simulink model "TrayectoriaStateflow"  (R2023b)
settings: Solver=FixedStepDiscrete  StartTime=0.0  StopTime=inf  FixedStep=0.01  RelTol=1e-3  EnableMultiTasking=on
settings Model: ExtModeTrigDuration=2  Creator=Usuario_UMA  LastModifiedBy=Usuario_UMA
settings OptimizationCC: EnhancedBackFolding=on  PassReuseOutputArgsAs=Individual arguments  ZeroExternalMemoryAtStartup=off  ZeroInternalMemoryAtStartup=off  MaxStackSize=64  OptimizeBlockOrder=speed  DifferentSizesBufferReuse=on  OptimizationCustomize=off  EfficientTunableParamExpr=on
settings DebuggingCC: ParameterTunabilityLossMsg=error
settings HardwareCC: ProdBitPerInt=16  ProdBitPerPointer=16  ProdBitPerSizeT=16  ProdBitPerPtrDiffT=16  ProdLargestAtomicFloat=None  ProdWordSize=8  ProdHWDeviceType=Atmel->AVR
settings SFSimCC: MATLABDynamicMemAlloc=off
settings RTWCC: Description=Embedded Coder  SystemTargetFile=ert.tlc  HardwareBoard=Arduino Mega 2560  TemplateMakefile=ert_default_tmf  Toolchain=Arduino AVR  BuildConfiguration=Faster Runs
settings CodeAppCC: ForceParamTrailComments=on  IgnoreCustomStorageClasses=off  OperatorAnnotations=on  SimulinkDataObjDesc=on  SFDataObjDesc=on  InsertBlockDesc=on
settings ERTTargetCC: SupportContinuousTime=on  SupportVariableSizeSignals=on  ExtModeTransport=3  ExtModeStaticAlloc=on  ExtModeAutomaticAllocSize=off  ExtModeStaticAllocSize=2048  ExtModeMexFile=ext_xcp  ExtModeIntrfLevel=Level2 - Open

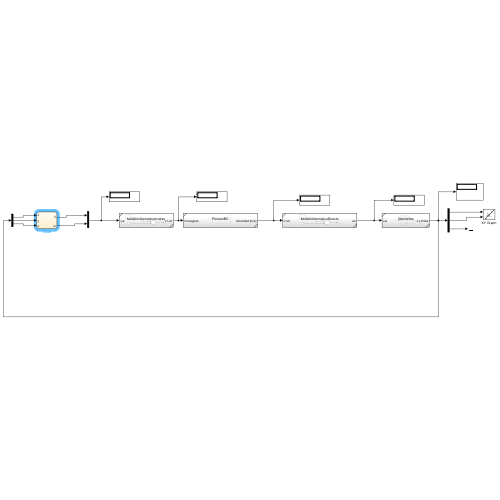
[thumbnail: Simulink's stored preview of the top-level diagram]
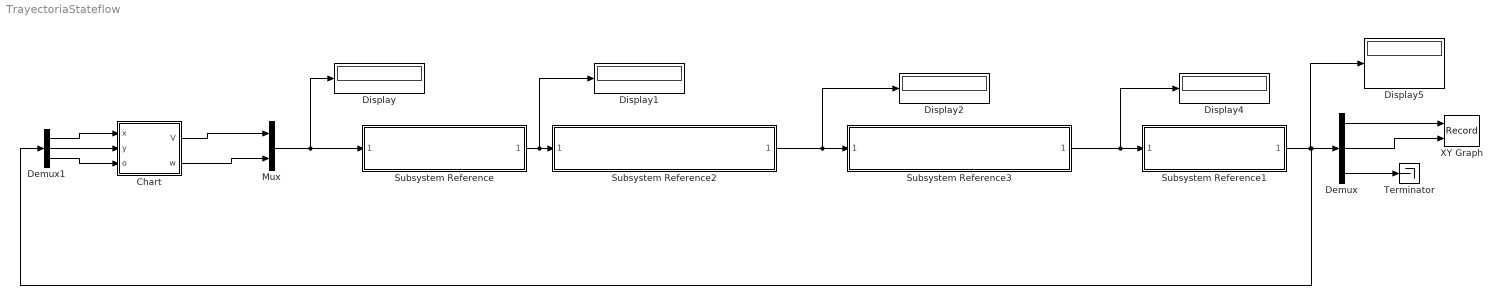
== system TrayectoriaStateflow ==
  Chart : Stateflow chart  TreatAsAtomicUnit=on
  Demux : Demux  Outputs=3
  Demux1 : Demux  Outputs=3
  Display{,1..2,4..5} (5 alike) : Display
  Mux : Mux  Inputs=2
  Subsystem Reference : Subsystem  ReferencedSubsystem=ModelocinematicoInverso
  Subsystem Reference1 : Subsystem  ReferencedSubsystem=Odometria
  Subsystem Reference2 : Subsystem  ReferencedSubsystem=PieroenBC
  Subsystem Reference3 : Subsystem  ReferencedSubsystem=ModelocinematicoDirecto
  Terminator : Terminator
  XY Graph : Record  FileSettingsInternal="{\"entries\":[{\"content\":{\"excelSettings\":{\"content\":{},\"type\":\"Streamout.ExcelSettings\"}},\"type\":\"Streamout.FileSettingStorage\",\"uuid\":\"\"}],\"packageUris\":[\"http:\\/\\/schema.mathworks.com\\/mf0\\/streamout_blocks\\/R2020a\"],\"version\":\"1.0\"}"  Layout=[1 1]  SignalsInternal="{\"entries\":[{\"content\":{},\"type\":\"RecordBlkView.InputSignals\",\"uuid\":\"\"}],\"packageUris\":[\"http:\\/\\/schema.mathworks.com\\/mf0\\/streamout_blocks\\/R2020a\"],\"version\":\"1.0\"}"  VisualizationBindings="{\"xyplotplugin\":{\"info\":[{\"series\":[],\"subplotID\":1}]}}"  CompatibilityTag=XY
  wires:
  Subsystem Reference/1 -> Display1/1, Subsystem Reference2/1
  Mux/1 -> Display/1, Subsystem Reference/1
  Subsystem Reference2/1 -> Display2/1, Subsystem Reference3/1
  Subsystem Reference3/1 -> Display4/1, Subsystem Reference1/1
  Subsystem Reference1/1 -> Display5/1, Demux1/1, Demux/1
  Demux/1 -> XY Graph/1
  Demux/2 -> XY Graph/2
  Demux/3 -> Terminator/1
  Chart/1(V) -> Mux/1
  Chart/2(w) -> Mux/2
  Demux1/1 -> Chart/1(x)
  Demux1/2 -> Chart/2(y)
  Demux1/3 -> Chart/3(o)

== stateflow chart TrayectoriaStateflow/Chart ==
  state Inicio
    entry:
    V = 0;
    w = 0;
  state Marcha
    entry:
    V = 0.205;
    w = 0;
  state Giroizquierda
    entry:
    V = 0.1;
    w = pi/4;
  state Recto12
    entry:
    V = 0.205;
    w = 0;
  state Giroderecha
    entry:
    V = 0.1;
    w = -pi/4;
  state Recto1
    entry:
    V = 0.205;
    w = 0;
  state GiroIzquierda1
    entry:
    V = 0.1;
    w = pi/4;
  state Recto4
    entry:
    V = 0.205;
    w = 0;
  state Paro
    entry:
    V = 0;
    w = 0;
  (default) -> Inicio
  Inicio -> Marcha : after(1,sec)
  Marcha -> Giroizquierda : [x>2.1]
  Recto1 -> GiroIzquierda1 : [x>3]
  Giroizquierda -> Recto12 : [o>pi/2]
  Recto4 -> Paro : [y>14]
  Recto12 -> Giroderecha : [y>12]
  Giroderecha -> Recto1 : [o>0]
  GiroIzquierda1 -> Recto4 : [o>pi/2]
  data: V output; w output; x input; y input; o input
